simulink library "monroe_library"  (R2012b)
settings: Solver=ode45  StartTime=0.0  StopTime=10.0  RelTol=1e-3
values from neighbouring files (symbols this model uses):
  input_bit_width = ', num2str(input_bit_width))    [fft_direct_draw.m]
undefined symbols (not defined in the file or in its folder): gcbh, xlBlockLoadCallback
libraries: xbsIndex_r4 x1880, monroe_library x159, casper_library x13, xps_library x1
(part 9 of 43)

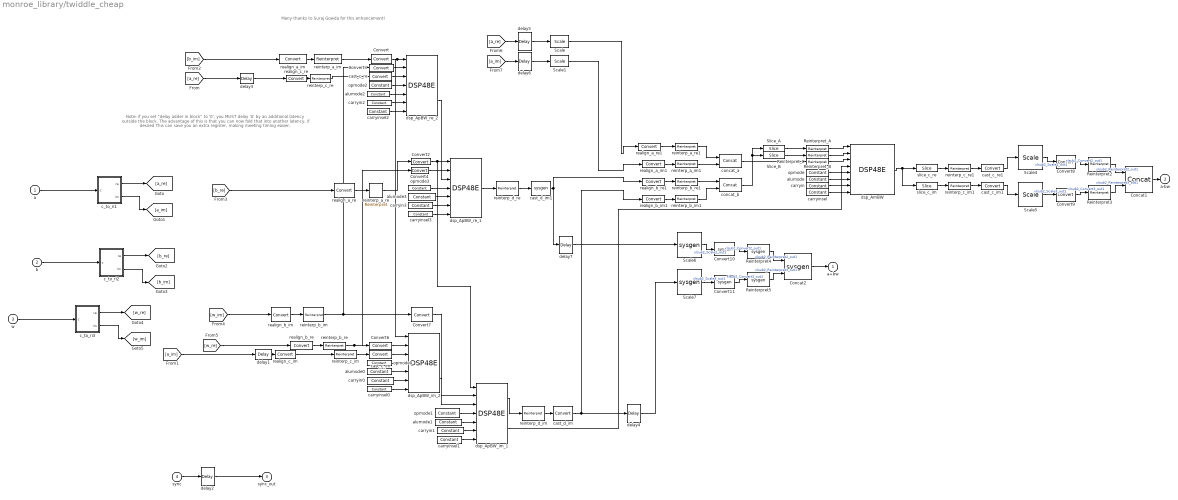
== system monroe_library/twiddle_cheap ==
  note: Note: if you set "delay adder in block" to '0', you MUST
      | delay 'A' by an additional latency outside the block.  The advantage of this
      | is that you can now fold that into another latency, if desired
      | This can save you an extra register, making meeting timing easier.
  note: Many thanks to Suraj Gowda for this enhancement!
  a : Inport
  b : Inport  Port=2
  w : Inport  Port=3
  sync : Inport  Port=4
  Concat1 : xbsIndex_r4/Concat  num_inputs=2  dbl_ovrd=off  block_type=concat
  Concat2 : S-Function  LoadFcn=xlBlockLoadCallback(gcbh);  FunctionName=sysgen  Parameters=ptable_  EnableBusSupport=off  mask(Xilinx Bus Concatenator Block){infoedit=Concatenates two or more inputs.  Output will be cast to an unsigned value with the binary point at zero., num_inputs=2, dbl_ovrd_sgadvanced=, dbl_ovrd=off, has_advanced_control=0, sggui_pos=-1,-1,-1,-1, block_type=concat, block_version=, sg_icon_stat=60,60,2,1,white,blue,0,16398980,right,,[ ],[ ], sg_mask_display=|, sg_list_contents=, sg_blockgui_xml=}
      mask sg_mask_display=|
      | fprintf('','COMMENT: begin icon graphics');
      | patch([0 60 60 0 0 ],[0 0 60 60 0 ],[0.77 0.82 0.91 ]);
      | plot([0 60 60 0 0 ],[0 0 60 60 0 ]);
      | patch([12.2 23.76 31.76 39.76 47.76 31.76 20.2 12.2 ],[38.88 38.88 46.88 38.88 46.88 46.88 46.88 38.88 ],[1 1 1 ]);
      | patch([20.2 31.76 23.76 12.2 20.2 ],[30.88 30.88 38.88 38.88 30.88 ],[0.931 0.946 0.973 ]);
      | patch([12.2 23.76 31.76 20.2 12.2 ],[22.88 22.88 30.88 30.88 22.88 ],[1 1 1 ]);
      | patch([20.2 47.76 39.76 31.76 23.76 12.2 20.2 ],[14.88 14.88 22.88 14.88 22.88 22.88 14.88 ],[0.931 0.946 0.973 ]);
      | fprintf('','COMMENT: end icon graphics');
      | fprintf('','COMMENT: begin icon text');
      | color('black');port_label('input',1,'hi');
      | color('black');port_label('input',2,'lo');
      |
      | color('black');disp('\fontsize{20}\}','texmode','on');
      | fprintf('','COMMENT: end icon text');
      mask prompts: infoedit ""; num_inputs "Number of inputs"; dbl_ovrd_sgadvanced ""; dbl_ovrd "Override with doubles"; has_advanced_control ""; sggui_pos ""; block_type ""; block_version ""; sg_icon_stat ""; sg_mask_display ""; sg_list_contents ""; sg_blockgui_xml ""
      mask help: Concatenates two or more inputs. Output will be cast to an unsigned value with the binary point at zero.
      mask init: same as monroe_library/double_delay_bram_external_counter/Concat1
      settings: CopyFcn=xlBlockMoveCallback(gcbh);  DeleteFcn=xlDestroyGui(gcbh);  ModelCloseFcn=xlDestroyGui(gcbh);  PreSaveFcn=xlBlockPreSaveCallback(gcbh);  PostSaveFcn=xlBlockPostSaveCallback(gcbh);  DestroyFcn=xlDestroyGui(gcbh);  OpenFcn=xlOpenGui(gcbh, 'concat_gui.xml', @xlmagicenablement, -1)  CloseFcn=xlDestroyGui(gcbh);  MoveFcn=xlBlockMoveCallback(gcbh);
      mask Help: eval('');xlDoc('-book','sysgen','-topic','Concat');
      mask Display:
      | fprintf('','COMMENT: begin icon graphics');
      | patch([0 60 60 0 0 ],[0 0 60 60 0 ],[0.77 0.82 0.91 ]);
      | plot([0 60 60 0 0 ],[0 0 60 60 0 ]);
      | patch([12.2 23.76 31.76 39.76 47.76 31.76 20.2 12.2 ],[38.88 38.88 46.88 38.88 46.88 46.88 46.88 38.88 ],[1 1 1 ]);
      | patch([20.2 31.76 23.76 12.2 20.2 ],[30.88 30.88 38.88 38.88 30.88 ],[0.931 0.946 0.973 ]);
      | patch([12.2 23.76 31.76 20.2 12.2 ],[22.88 22.88 30.88 30.88 22.88 ],[1 1 1 ]);
      | patch([20.2 47.76 39.76 31.76 23.76 12.2 20.2 ],[14.88 14.88 22.88 14.88 22.88 22.88 14.88 ],[0.931 0.946 0.973 ]);
      | fprintf('','COMMENT: end icon graphics');
      | fprintf('','COMMENT: begin icon text');
      | color('black');port_label('input',1,'hi');
      | color('black');port_label('input',2,'lo');
      | 
      | color('black');disp('\fontsize{20}\}','texmode','on');
      | fprintf('','COMMENT: end icon text');
  Convert : xbsIndex_r4/Convert  arith_type="Signed  (2's comp)"  n_bits=30  bin_pt=0  quantization=Truncate  overflow=Wrap  en=off  latency=0  dbl_ovrd=off  pipeline=on  block_type=convert
      settings: block_version=11.4
  Convert10 : S-Function  LoadFcn=xlBlockLoadCallback(gcbh);  FunctionName=sysgen  Parameters=ptable_  EnableBusSupport=off  mask(Xilinx Type Converter Block){infoedit=Hardware notes: rounding and saturating require hardware resources; truncating and wrapping do not., arith_type_sgadvanced=, arith_type=Signed  (2's comp), n_bits=out_n_bits, bin_pt=out_n_bits-1, quantization_sgadvanced=, quantization=Truncate, overflow_sgadvanced=, overflow=Wrap, en_sgadvanced=, en=off, latency=0, dbl_ovrd_sgadvanced=, dbl_ovrd=off, pipeline_sgadvanced=, pipeline=off, xl_use_area_sgadvanced=, xl_use_area=off, xl_area=[0,0,0,0,0,0,0], has_advanced_control=0, sggui_pos=-1,-1,-1,-1, block_type=convert, block_version=, sg_icon_stat=45,30,1,1,white,blue,0,edca21da,right,,[ ],[ ], sg_mask_display=|, sg_list_contents=, sg_blockgui_xml=}
      mask sg_mask_display=|
      | fprintf('','COMMENT: begin icon graphics');
      | patch([0 45 45 0 0 ],[0 0 30 30 0 ],[0.77 0.82 0.91 ]);
      | plot([0 45 45 0 0 ],[0 0 30 30 0 ]);
      | patch([13.1 18.88 22.88 26.88 30.88 22.88 17.1 13.1 ],[19.44 19.44 23.44 19.44 23.44 23.44 23.44 19.44 ],[1 1 1 ]);
      | patch([17.1 22.88 18.88 13.1 17.1 ],[15.44 15.44 19.44 19.44 15.44 ],[0.931 0.946 0.973 ]);
      | patch([13.1 18.88 22.88 17.1 13.1 ],[11.44 11.44 15.44 15.44 11.44 ],[1 1 1 ]);
      | patch([17.1 30.88 26.88 22.88 18.88 13.1 17.1 ],[7.44 7.44 11.44 7.44 11.44 11.44 7.44 ],[0.931 0.946 0.973 ]);
      | fprintf('','COMMENT: end icon graphics');
      | fprintf('','COMMENT: begin icon text');
      |
      | color('black');port_label('output',1,'cast');
      | fprintf('','COMMENT: end icon text');
      mask prompts: infoedit ""; arith_type_sgadvanced ""; arith_type "Type"; n_bits "Number of bits"; bin_pt "Binary point"; quantization_sgadvanced ""; overflow_sgadvanced ""; en_sgadvanced ""; en "Provide enable port"; dbl_ovrd_sgadvanced ""; dbl_ovrd "Override with doubles"; pipeline_sgadvanced ""; pipeline "Pipeline for maximum performance"; xl_use_area_sgadvanced ""; xl_use_area "Define FPGA area for resource estimation"; xl_area "FPGA area [slices, FFs, BRAMs, LUTs, IOBs, emb. mults, TBUFs]"; has_advanced_control ""; sggui_pos ""; block_type ""; block_version ""; sg_icon_stat ""; sg_mask_display ""; sg_list_contents ""; sg_blockgui_xml ""
      mask help: Hardware notes: rounding and saturating require hardware resources; truncating and wrapping do not.
      mask init: same as monroe_library/dsp48e_mult_add_pcin/Convert
      settings: CopyFcn=xlBlockMoveCallback(gcbh);  DeleteFcn=xlDestroyGui(gcbh);  ModelCloseFcn=xlDestroyGui(gcbh);  PreSaveFcn=xlBlockPreSaveCallback(gcbh);  PostSaveFcn=xlBlockPostSaveCallback(gcbh);  DestroyFcn=xlDestroyGui(gcbh);  OpenFcn=xlOpenGui(gcbh, 'convert_gui.xml', @convertenablement, -1)  CloseFcn=xlDestroyGui(gcbh);  MoveFcn=xlBlockMoveCallback(gcbh);
      mask Help: eval('');xlDoc('-book','sysgen','-topic','Convert');
      mask TypeOptions arith_type: Boolean | Signed  (2's comp) | Unsigned
      mask TypeOptions quantization: Truncate | Round  (unbiased: +/- Inf) | Round  (unbiased: Even Values)
      mask TypeOptions overflow: Wrap | Saturate | Flag as error
      mask Display:
      | fprintf('','COMMENT: begin icon graphics');
      | patch([0 45 45 0 0 ],[0 0 30 30 0 ],[0.77 0.82 0.91 ]);
      | plot([0 45 45 0 0 ],[0 0 30 30 0 ]);
      | patch([13.1 18.88 22.88 26.88 30.88 22.88 17.1 13.1 ],[19.44 19.44 23.44 19.44 23.44 23.44 23.44 19.44 ],[1 1 1 ]);
      | patch([17.1 22.88 18.88 13.1 17.1 ],[15.44 15.44 19.44 19.44 15.44 ],[0.931 0.946 0.973 ]);
      | patch([13.1 18.88 22.88 17.1 13.1 ],[11.44 11.44 15.44 15.44 11.44 ],[1 1 1 ]);
      | patch([17.1 30.88 26.88 22.88 18.88 13.1 17.1 ],[7.44 7.44 11.44 7.44 11.44 11.44 7.44 ],[0.931 0.946 0.973 ]);
      | fprintf('','COMMENT: end icon graphics');
      | fprintf('','COMMENT: begin icon text');
      | 
      | color('black');port_label('output',1,'cast');
      | fprintf('','COMMENT: end icon text');
  Convert11 : S-Function  LoadFcn=xlBlockLoadCallback(gcbh);  FunctionName=sysgen  Parameters=ptable_  EnableBusSupport=off  mask(Xilinx Type Converter Block){infoedit=Hardware notes: rounding and saturating require hardware resources; truncating and wrapping do not., arith_type_sgadvanced=, arith_type=Signed  (2's comp), n_bits=out_n_bits, bin_pt=out_n_bits-1, quantization_sgadvanced=, quantization=Truncate, overflow_sgadvanced=, overflow=Wrap, en_sgadvanced=, en=off, latency=0, dbl_ovrd_sgadvanced=, dbl_ovrd=off, pipeline_sgadvanced=, pipeline=off, xl_use_area_sgadvanced=, xl_use_area=off, xl_area=[0,0,0,0,0,0,0], has_advanced_control=0, sggui_pos=-1,-1,-1,-1, block_type=convert, block_version=, sg_icon_stat=45,30,1,1,white,blue,0,edca21da,right,,[ ],[ ], sg_mask_display=|, sg_list_contents=, sg_blockgui_xml=}
      mask sg_mask_display=|
      | fprintf('','COMMENT: begin icon graphics');
      | patch([0 45 45 0 0 ],[0 0 30 30 0 ],[0.77 0.82 0.91 ]);
      | plot([0 45 45 0 0 ],[0 0 30 30 0 ]);
      | patch([13.1 18.88 22.88 26.88 30.88 22.88 17.1 13.1 ],[19.44 19.44 23.44 19.44 23.44 23.44 23.44 19.44 ],[1 1 1 ]);
      | patch([17.1 22.88 18.88 13.1 17.1 ],[15.44 15.44 19.44 19.44 15.44 ],[0.931 0.946 0.973 ]);
      | patch([13.1 18.88 22.88 17.1 13.1 ],[11.44 11.44 15.44 15.44 11.44 ],[1 1 1 ]);
      | patch([17.1 30.88 26.88 22.88 18.88 13.1 17.1 ],[7.44 7.44 11.44 7.44 11.44 11.44 7.44 ],[0.931 0.946 0.973 ]);
      | fprintf('','COMMENT: end icon graphics');
      | fprintf('','COMMENT: begin icon text');
      |
      | color('black');port_label('output',1,'cast');
      | fprintf('','COMMENT: end icon text');
      mask prompts: infoedit ""; arith_type_sgadvanced ""; arith_type "Type"; n_bits "Number of bits"; bin_pt "Binary point"; quantization_sgadvanced ""; overflow_sgadvanced ""; en_sgadvanced ""; en "Provide enable port"; dbl_ovrd_sgadvanced ""; dbl_ovrd "Override with doubles"; pipeline_sgadvanced ""; pipeline "Pipeline for maximum performance"; xl_use_area_sgadvanced ""; xl_use_area "Define FPGA area for resource estimation"; xl_area "FPGA area [slices, FFs, BRAMs, LUTs, IOBs, emb. mults, TBUFs]"; has_advanced_control ""; sggui_pos ""; block_type ""; block_version ""; sg_icon_stat ""; sg_mask_display ""; sg_list_contents ""; sg_blockgui_xml ""
      mask help: Hardware notes: rounding and saturating require hardware resources; truncating and wrapping do not.
      mask init: same as monroe_library/dsp48e_mult_add_pcin/Convert
      settings: CopyFcn=xlBlockMoveCallback(gcbh);  DeleteFcn=xlDestroyGui(gcbh);  ModelCloseFcn=xlDestroyGui(gcbh);  PreSaveFcn=xlBlockPreSaveCallback(gcbh);  PostSaveFcn=xlBlockPostSaveCallback(gcbh);  DestroyFcn=xlDestroyGui(gcbh);  OpenFcn=xlOpenGui(gcbh, 'convert_gui.xml', @convertenablement, -1)  CloseFcn=xlDestroyGui(gcbh);  MoveFcn=xlBlockMoveCallback(gcbh);
      mask Help: eval('');xlDoc('-book','sysgen','-topic','Convert');
      mask TypeOptions arith_type: Boolean | Signed  (2's comp) | Unsigned
      mask TypeOptions quantization: Truncate | Round  (unbiased: +/- Inf) | Round  (unbiased: Even Values)
      mask TypeOptions overflow: Wrap | Saturate | Flag as error
      mask Display:
      | fprintf('','COMMENT: begin icon graphics');
      | patch([0 45 45 0 0 ],[0 0 30 30 0 ],[0.77 0.82 0.91 ]);
      | plot([0 45 45 0 0 ],[0 0 30 30 0 ]);
      | patch([13.1 18.88 22.88 26.88 30.88 22.88 17.1 13.1 ],[19.44 19.44 23.44 19.44 23.44 23.44 23.44 19.44 ],[1 1 1 ]);
      | patch([17.1 22.88 18.88 13.1 17.1 ],[15.44 15.44 19.44 19.44 15.44 ],[0.931 0.946 0.973 ]);
      | patch([13.1 18.88 22.88 17.1 13.1 ],[11.44 11.44 15.44 15.44 11.44 ],[1 1 1 ]);
      | patch([17.1 30.88 26.88 22.88 18.88 13.1 17.1 ],[7.44 7.44 11.44 7.44 11.44 11.44 7.44 ],[0.931 0.946 0.973 ]);
      | fprintf('','COMMENT: end icon graphics');
      | fprintf('','COMMENT: begin icon text');
      | 
      | color('black');port_label('output',1,'cast');
      | fprintf('','COMMENT: end icon text');
  Convert2 : xbsIndex_r4/Convert  arith_type="Signed  (2's comp)"  n_bits=30  bin_pt=0  quantization=Truncate  overflow=Wrap  en=off  latency=0  dbl_ovrd=off  pipeline=on  block_type=convert
      settings: block_version=11.4
  Convert{3..4,6..7} (4 alike) : xbsIndex_r4/Convert  arith_type="Signed  (2's comp)"  n_bits=18  bin_pt=0  quantization=Truncate  overflow=Wrap  en=off  latency=0  dbl_ovrd=off  pipeline=on  block_type=convert
      settings: block_version=11.4
  Convert8 : xbsIndex_r4/Convert  arith_type="Signed  (2's comp)"  n_bits=out_n_bits  bin_pt=out_n_bits-1  quantization=Truncate  overflow=Wrap  en=off  latency=0  dbl_ovrd=off  pipeline=off  block_type=convert
  Convert9 : xbsIndex_r4/Convert  arith_type="Signed  (2's comp)"  n_bits=out_n_bits  bin_pt=out_n_bits-1  quantization=Truncate  overflow=Wrap  en=off  latency=0  dbl_ovrd=off  pipeline=off  block_type=convert
  Reinterpret2 : xbsIndex_r4/Reinterpret  force_arith_type=on  arith_type=Unsigned  force_bin_pt=on  bin_pt=0  block_type=reinterpret
      settings: infoedit="Changes signal type without altering the binary representation.   You can changed the signal between signed and unsigned, and relocate the binary point.<br><br>Hardware notes: In hardware this block costs nothing.<br><br>Example:  Suppose the input is 6 bits wide, signed, with 2 fractional bits, and the output is forced to unsigned with 0 fractional bits.  Then an input of -2.0 (1110.00 in binary 2's complement) becomes an output of 56 (111000 in binary)."
  Reinterpret3 : xbsIndex_r4/Reinterpret  force_arith_type=on  arith_type=Unsigned  force_bin_pt=on  bin_pt=0  block_type=reinterpret
      settings: infoedit="Changes signal type without altering the binary representation.   You can changed the signal between signed and unsigned, and relocate the binary point.<br><br>Hardware notes: In hardware this block costs nothing.<br><br>Example:  Suppose the input is 6 bits wide, signed, with 2 fractional bits, and the output is forced to unsigned with 0 fractional bits.  Then an input of -2.0 (1110.00 in binary 2's complement) becomes an output of 56 (111000 in binary)."
  Reinterpret4 : S-Function  LoadFcn=xlBlockLoadCallback(gcbh);  FunctionName=sysgen  Parameters=ptable_  EnableBusSupport=off  mask(Xilinx Type Reinterpreter Block){infoedit=Changes signal type without altering the binary representation.   You can changed the signal between signed and unsigned, and relocate the binary point.<br><br>Hardware notes: In hardware this block costs nothing.<br><br>Example:  Suppose the input is 6 bits wide, signed, with 2 fractional bits, and the output is forced to unsigned with 0 fractional bits.  Then an input of -2.0 (1110.00 in binary 2's complement) becomes an output of 56 (111000 in binary)., force_arith_type_sgadvanced=, force_arith_type=on, arith_type_sgadvanced=, arith_type=Unsigned, force_bin_pt_sgadvanced=, force_bin_pt=on, bin_pt=0, has_advanced_control=0, sggui_pos=-1,-1,-1,-1, block_type=reinterpret, block_version=, sg_icon_stat=50,32,1,1,white,blue,0,6b04d0b0,right,,[ ],[ ], sg_mask_display=|, sg_list_contents=, sg_blockgui_xml=}
      mask sg_mask_display=|
      | fprintf('','COMMENT: begin icon graphics');
      | patch([0 50 50 0 0 ],[0 0 32 32 0 ],[0.77 0.82 0.91 ]);
      | plot([0 50 50 0 0 ],[0 0 32 32 0 ]);
      | patch([16.1 21.88 25.88 29.88 33.88 25.88 20.1 16.1 ],[20.44 20.44 24.44 20.44 24.44 24.44 24.44 20.44 ],[1 1 1 ]);
      | patch([20.1 25.88 21.88 16.1 20.1 ],[16.44 16.44 20.44 20.44 16.44 ],[0.931 0.946 0.973 ]);
      | patch([16.1 21.88 25.88 20.1 16.1 ],[12.44 12.44 16.44 16.44 12.44 ],[1 1 1 ]);
      | patch([20.1 33.88 29.88 25.88 21.88 16.1 20.1 ],[8.44 8.44 12.44 8.44 12.44 12.44 8.44 ],[0.931 0.946 0.973 ]);
      | fprintf('','COMMENT: end icon graphics');
      | fprintf('','COMMENT: begin icon text');
      |
      |
      | color('black');disp('reinterpret');
      | fprintf('','COMMENT: end icon text');
      mask prompts: infoedit ""; force_arith_type_sgadvanced ""; force_arith_type "Force Arithmetic Type"; arith_type_sgadvanced ""; arith_type "Output Arithmetic Type"; force_bin_pt_sgadvanced ""; force_bin_pt "Force Binary Point"; bin_pt "Output Binary Point"; has_advanced_control ""; sggui_pos ""; block_type ""; block_version ""; sg_icon_stat ""; sg_mask_display ""; sg_list_contents ""; sg_blockgui_xml ""
      mask help:
      | Changes signal type without altering the binary representation.   You can changed the signal between signed and unsigned, and relocate the binary point.
      |
      | Hardware notes: In hardware this block costs nothing.
      |
      | Example:  Suppose the input is 6 bits wide, signed, with 2 fractional bits, and the output is forced to unsigned with 0 fractional bits.  Then an input of -2.0 (1110.00 in binary 2's complement) becomes an output of 56 (111000 in binary).
      mask init:
      | try
      |   tmp_gcb = gcb;
      |   tmp_gcbh = gcbh;
      |   if (strcmp('SysGenIndex',get_param(bdroot(tmp_gcbh),'tag')) && ~isempty(regexp(bdroot(tmp_gcb), '^xbs', 'once')))
      |     return;
      |   end;
      |   xlMungeMaskParams;
      |   block_config = 'sysgen_blockset:Reinterpret_config';
      | 
      |   block_type='reinterpret';
      | 
      |   serialized_declarations = '{''arith_type''=>''Int'',''bin_pt''=>''Int'',''force_arith_type''=>''Bool'',''force_bin_pt''=>''Bool'',''block_type''=>''String''}';
      |   ptable_ = xlblockprep(get_param(tmp_gcb, 'MaskWSVariables'));
      |   try
      |     xlBlockMoveCallback(tmp_gcbh);
      |   catch 
      |      clear global xl_updateicon_recursion_guard;
      |   end;
      | catch
      |   global dbgsysgen;
      |   if(~isempty(dbgsysgen) && dbgsysgen)
      |     e = regexprep(lasterr, '\n', '\nError: ');
      |     disp(['Error: While running MaskInit code on block ' tmp_gcb ': ' e]);
      |     error(e);
      |   end
      | end
      settings: CopyFcn=xlBlockMoveCallback(gcbh);  DeleteFcn=xlDestroyGui(gcbh);  ModelCloseFcn=xlDestroyGui(gcbh);  PreSaveFcn=xlBlockPreSaveCallback(gcbh);  PostSaveFcn=xlBlockPostSaveCallback(gcbh);  DestroyFcn=xlDestroyGui(gcbh);  OpenFcn=xlOpenGui(gcbh, 'reinterpret_gui.xml', @reinterpretenablement, -1)  CloseFcn=xlDestroyGui(gcbh);  MoveFcn=xlBlockMoveCallback(gcbh);
      mask Help: eval('');xlDoc('-book','sysgen','-topic','Reinterpret');
      mask TypeOptions arith_type: Unsigned | Signed  (2's comp)
      mask Display:
      | fprintf('','COMMENT: begin icon graphics');
      | patch([0 50 50 0 0 ],[0 0 32 32 0 ],[0.77 0.82 0.91 ]);
      | plot([0 50 50 0 0 ],[0 0 32 32 0 ]);
      | patch([16.1 21.88 25.88 29.88 33.88 25.88 20.1 16.1 ],[20.44 20.44 24.44 20.44 24.44 24.44 24.44 20.44 ],[1 1 1 ]);
      | patch([20.1 25.88 21.88 16.1 20.1 ],[16.44 16.44 20.44 20.44 16.44 ],[0.931 0.946 0.973 ]);
      | patch([16.1 21.88 25.88 20.1 16.1 ],[12.44 12.44 16.44 16.44 12.44 ],[1 1 1 ]);
      | patch([20.1 33.88 29.88 25.88 21.88 16.1 20.1 ],[8.44 8.44 12.44 8.44 12.44 12.44 8.44 ],[0.931 0.946 0.973 ]);
      | fprintf('','COMMENT: end icon graphics');
      | fprintf('','COMMENT: begin icon text');
      | 
      | 
      | color('black');disp('reinterpret');
      | fprintf('','COMMENT: end icon text');
  Reinterpret5 : S-Function  LoadFcn=xlBlockLoadCallback(gcbh);  FunctionName=sysgen  Parameters=ptable_  EnableBusSupport=off  mask(Xilinx Type Reinterpreter Block){infoedit=Changes signal type without altering the binary representation.   You can changed the signal between signed and unsigned, and relocate the binary point.<br><br>Hardware notes: In hardware this block costs nothing.<br><br>Example:  Suppose the input is 6 bits wide, signed, with 2 fractional bits, and the output is forced to unsigned with 0 fractional bits.  Then an input of -2.0 (1110.00 in binary 2's complement) becomes an output of 56 (111000 in binary)., force_arith_type_sgadvanced=, force_arith_type=on, arith_type_sgadvanced=, arith_type=Unsigned, force_bin_pt_sgadvanced=, force_bin_pt=on, bin_pt=0, has_advanced_control=0, sggui_pos=-1,-1,-1,-1, block_type=reinterpret, block_version=, sg_icon_stat=50,32,1,1,white,blue,0,6b04d0b0,right,,[ ],[ ], sg_mask_display=|, sg_list_contents=, sg_blockgui_xml=}
      mask sg_mask_display=|
      | fprintf('','COMMENT: begin icon graphics');
      | patch([0 50 50 0 0 ],[0 0 32 32 0 ],[0.77 0.82 0.91 ]);
      | plot([0 50 50 0 0 ],[0 0 32 32 0 ]);
      | patch([16.1 21.88 25.88 29.88 33.88 25.88 20.1 16.1 ],[20.44 20.44 24.44 20.44 24.44 24.44 24.44 20.44 ],[1 1 1 ]);
      | patch([20.1 25.88 21.88 16.1 20.1 ],[16.44 16.44 20.44 20.44 16.44 ],[0.931 0.946 0.973 ]);
      | patch([16.1 21.88 25.88 20.1 16.1 ],[12.44 12.44 16.44 16.44 12.44 ],[1 1 1 ]);
      | patch([20.1 33.88 29.88 25.88 21.88 16.1 20.1 ],[8.44 8.44 12.44 8.44 12.44 12.44 8.44 ],[0.931 0.946 0.973 ]);
      | fprintf('','COMMENT: end icon graphics');
      | fprintf('','COMMENT: begin icon text');
      |
      |
      | color('black');disp('reinterpret');
      | fprintf('','COMMENT: end icon text');
      mask prompts: infoedit ""; force_arith_type_sgadvanced ""; force_arith_type "Force Arithmetic Type"; arith_type_sgadvanced ""; arith_type "Output Arithmetic Type"; force_bin_pt_sgadvanced ""; force_bin_pt "Force Binary Point"; bin_pt "Output Binary Point"; has_advanced_control ""; sggui_pos ""; block_type ""; block_version ""; sg_icon_stat ""; sg_mask_display ""; sg_list_contents ""; sg_blockgui_xml ""
      mask help:
      | Changes signal type without altering the binary representation.   You can changed the signal between signed and unsigned, and relocate the binary point.
      |
      | Hardware notes: In hardware this block costs nothing.
      |
      | Example:  Suppose the input is 6 bits wide, signed, with 2 fractional bits, and the output is forced to unsigned with 0 fractional bits.  Then an input of -2.0 (1110.00 in binary 2's complement) becomes an output of 56 (111000 in binary).
      mask init: same as monroe_library/twiddle_cheap/Reinterpret4
      settings: CopyFcn=xlBlockMoveCallback(gcbh);  DeleteFcn=xlDestroyGui(gcbh);  ModelCloseFcn=xlDestroyGui(gcbh);  PreSaveFcn=xlBlockPreSaveCallback(gcbh);  PostSaveFcn=xlBlockPostSaveCallback(gcbh);  DestroyFcn=xlDestroyGui(gcbh);  OpenFcn=xlOpenGui(gcbh, 'reinterpret_gui.xml', @reinterpretenablement, -1)  CloseFcn=xlDestroyGui(gcbh);  MoveFcn=xlBlockMoveCallback(gcbh);
      mask Help: eval('');xlDoc('-book','sysgen','-topic','Reinterpret');
      mask TypeOptions arith_type: Unsigned | Signed  (2's comp)
      mask Display:
      | fprintf('','COMMENT: begin icon graphics');
      | patch([0 50 50 0 0 ],[0 0 32 32 0 ],[0.77 0.82 0.91 ]);
      | plot([0 50 50 0 0 ],[0 0 32 32 0 ]);
      | patch([16.1 21.88 25.88 29.88 33.88 25.88 20.1 16.1 ],[20.44 20.44 24.44 20.44 24.44 24.44 24.44 20.44 ],[1 1 1 ]);
      | patch([20.1 25.88 21.88 16.1 20.1 ],[16.44 16.44 20.44 20.44 16.44 ],[0.931 0.946 0.973 ]);
      | patch([16.1 21.88 25.88 20.1 16.1 ],[12.44 12.44 16.44 16.44 12.44 ],[1 1 1 ]);
      | patch([20.1 33.88 29.88 25.88 21.88 16.1 20.1 ],[8.44 8.44 12.44 8.44 12.44 12.44 8.44 ],[0.931 0.946 0.973 ]);
      | fprintf('','COMMENT: end icon graphics');
      | fprintf('','COMMENT: begin icon text');
      | 
      | 
      | color('black');disp('reinterpret');
      | fprintf('','COMMENT: end icon text');
  Reinterpret_A : xbsIndex_r4/Reinterpret  force_arith_type=on  arith_type="Signed  (2's comp)"  force_bin_pt=on  bin_pt=0  block_type=reinterpret
      settings: infoedit="Changes signal type without altering the binary representation.   You can changed the signal between signed and unsigned, and relocate the binary point.<br><br>Hardware notes: In hardware this block costs nothing.<br><br>Example:  Suppose the input is 6 bits wide, signed, with 2 fractional bits, and the output is forced to unsigned with 0 fractional bits.  Then an input of -2.0 (1110.00 in binary 2's complement) becomes an output of 56 (111000 in binary)."  block_version=10.1.3
  Reinterpret_B : xbsIndex_r4/Reinterpret  force_arith_type=on  arith_type="Signed  (2's comp)"  force_bin_pt=on  bin_pt=0  block_type=reinterpret
      settings: infoedit="Changes signal type without altering the binary representation.   You can changed the signal between signed and unsigned, and relocate the binary point.<br><br>Hardware notes: In hardware this block costs nothing.<br><br>Example:  Suppose the input is 6 bits wide, signed, with 2 fractional bits, and the output is forced to unsigned with 0 fractional bits.  Then an input of -2.0 (1110.00 in binary 2's complement) becomes an output of 56 (111000 in binary)."  block_version=10.1.3
  Reinterpret_C : xbsIndex_r4/Reinterpret  force_arith_type=on  arith_type="Signed  (2's comp)"  force_bin_pt=on  bin_pt=0  block_type=reinterpret
      settings: infoedit="Changes signal type without altering the binary representation.   You can changed the signal between signed and unsigned, and relocate the binary point.<br><br>Hardware notes: In hardware this block costs nothing.<br><br>Example:  Suppose the input is 6 bits wide, signed, with 2 fractional bits, and the output is forced to unsigned with 0 fractional bits.  Then an input of -2.0 (1110.00 in binary 2's complement) becomes an output of 56 (111000 in binary)."  block_version=10.1.3
  Scale : xbsIndex_r4/Scale  scale_factor=1  dbl_ovrd=off  block_type=scale
  Scale1 : xbsIndex_r4/Scale  scale_factor=1  dbl_ovrd=off  block_type=scale
  Scale4 : xbsIndex_r4/Scale  scale_factor=downshift_at_end*-1  dbl_ovrd=off  block_type=scale
  Scale5 : xbsIndex_r4/Scale  scale_factor=downshift_at_end*-1  dbl_ovrd=off  block_type=scale
  Scale6 : S-Function  LoadFcn=xlBlockLoadCallback(gcbh);  FunctionName=sysgen  Parameters=ptable_  EnableBusSupport=off  mask(Xilinx Input Scaler Block){infoedit=Scales input by a power of two by adjusting the binary point position.<br><br>Hardware notes: In hardware this block costs nothing., scale_factor=downshift_at_end*-1, dbl_ovrd_sgadvanced=, dbl_ovrd=off, has_advanced_control=0, sggui_pos=-1,-1,-1,-1, block_type=scale, block_version=, sg_icon_stat=55,56,1,1,white,blue,0,e7f93c29,right,,[ ],[ ], sg_mask_display=|, sg_list_contents=, sg_blockgui_xml=}
      mask sg_mask_display=|
      | fprintf('','COMMENT: begin icon graphics');
      | patch([0 55 55 0 0 ],[0 0 56 56 0 ],[0.77 0.82 0.91 ]);
      | plot([0 55 55 0 0 ],[0 0 56 56 0 ]);
      | patch([11.425 21.54 28.54 35.54 42.54 28.54 18.425 11.425 ],[35.77 35.77 42.77 35.77 42.77 42.77 42.77 35.77 ],[1 1 1 ]);
      | patch([18.425 28.54 21.54 11.425 18.425 ],[28.77 28.77 35.77 35.77 28.77 ],[0.931 0.946 0.973 ]);
      | patch([11.425 21.54 28.54 18.425 11.425 ],[21.77 21.77 28.77 28.77 21.77 ],[1 1 1 ]);
      | patch([18.425 42.54 35.54 28.54 21.54 11.425 18.425 ],[14.77 14.77 21.77 14.77 21.77 21.77 14.77 ],[0.931 0.946 0.973 ]);
      | fprintf('','COMMENT: end icon graphics');
      | fprintf('','COMMENT: begin icon text');
      |
      |
      | color('black');disp('\bf{2^{0}}','texmode','on');
      | fprintf('','COMMENT: end icon text');
      mask prompts: infoedit ""; scale_factor "Scale factor s (scale output by 2^s)"; dbl_ovrd_sgadvanced ""; dbl_ovrd "Override with doubles"; has_advanced_control ""; sggui_pos ""; block_type ""; block_version ""; sg_icon_stat ""; sg_mask_display ""; sg_list_contents ""; sg_blockgui_xml ""
      mask help:
      | Scales input by a power of two by adjusting the binary point position.
      |
      | Hardware notes: In hardware this block costs nothing.
      mask init:
      | try
      |   tmp_gcb = gcb;
      |   tmp_gcbh = gcbh;
      |   if (strcmp('SysGenIndex',get_param(bdroot(tmp_gcbh),'tag')) && ~isempty(regexp(bdroot(tmp_gcb), '^xbs', 'once')))
      |     return;
      |   end;
      |   xlMungeMaskParams;
      |   block_config = 'sysgen_blockset:Scale_config';
      | 
      |   block_type='scale';
      | 
      |   serialized_declarations = '{''dbl_ovrd''=>''Int'',''scale_factor''=>''Int'',''block_type''=>''String''}';
      |   xlscale_init();
      |   ptable_ = xlblockprep(get_param(tmp_gcb, 'MaskWSVariables'));
      |   try
      |     xlBlockMoveCallback(tmp_gcbh);
      |   catch 
      |      clear global xl_updateicon_recursion_guard;
      |   end;
      | catch
      |   global dbgsysgen;
      |   if(~isempty(dbgsysgen) && dbgsysgen)
      |     e = regexprep(lasterr, '\n', '\nError: ');
      |     disp(['Error: While running MaskInit code on block ' tmp_gcb ': ' e]);
      |     error(e);
      |   end
      | end
      settings: CopyFcn=xlBlockMoveCallback(gcbh);  DeleteFcn=xlDestroyGui(gcbh);  ModelCloseFcn=xlDestroyGui(gcbh);  PreSaveFcn=xlBlockPreSaveCallback(gcbh);  PostSaveFcn=xlBlockPostSaveCallback(gcbh);  DestroyFcn=xlDestroyGui(gcbh);  OpenFcn=xlOpenGui(gcbh, 'scale_gui.xml', @xlmagicenablement, -1)  CloseFcn=xlDestroyGui(gcbh);  MoveFcn=xlBlockMoveCallback(gcbh);
      mask Help: eval('');xlDoc('-book','sysgen','-topic','Scale');
      mask Display:
      | fprintf('','COMMENT: begin icon graphics');
      | patch([0 55 55 0 0 ],[0 0 56 56 0 ],[0.77 0.82 0.91 ]);
      | plot([0 55 55 0 0 ],[0 0 56 56 0 ]);
      | patch([11.425 21.54 28.54 35.54 42.54 28.54 18.425 11.425 ],[35.77 35.77 42.77 35.77 42.77 42.77 42.77 35.77 ],[1 1 1 ]);
      | patch([18.425 28.54 21.54 11.425 18.425 ],[28.77 28.77 35.77 35.77 28.77 ],[0.931 0.946 0.973 ]);
      | patch([11.425 21.54 28.54 18.425 11.425 ],[21.77 21.77 28.77 28.77 21.77 ],[1 1 1 ]);
      | patch([18.425 42.54 35.54 28.54 21.54 11.425 18.425 ],[14.77 14.77 21.77 14.77 21.77 21.77 14.77 ],[0.931 0.946 0.973 ]);
      | fprintf('','COMMENT: end icon graphics');
      | fprintf('','COMMENT: begin icon text');
      | 
      | 
      | color('black');disp('\bf{2^{0}}','texmode','on');
      | fprintf('','COMMENT: end icon text');
  Scale7 : S-Function  LoadFcn=xlBlockLoadCallback(gcbh);  FunctionName=sysgen  Parameters=ptable_  EnableBusSupport=off  mask(Xilinx Input Scaler Block){infoedit=Scales input by a power of two by adjusting the binary point position.<br><br>Hardware notes: In hardware this block costs nothing., scale_factor=downshift_at_end*-1, dbl_ovrd_sgadvanced=, dbl_ovrd=off, has_advanced_control=0, sggui_pos=-1,-1,-1,-1, block_type=scale, block_version=, sg_icon_stat=55,56,1,1,white,blue,0,e7f93c29,right,,[ ],[ ], sg_mask_display=|, sg_list_contents=, sg_blockgui_xml=}
      mask sg_mask_display=|
      | fprintf('','COMMENT: begin icon graphics');
      | patch([0 55 55 0 0 ],[0 0 56 56 0 ],[0.77 0.82 0.91 ]);
      | plot([0 55 55 0 0 ],[0 0 56 56 0 ]);
      | patch([11.425 21.54 28.54 35.54 42.54 28.54 18.425 11.425 ],[35.77 35.77 42.77 35.77 42.77 42.77 42.77 35.77 ],[1 1 1 ]);
      | patch([18.425 28.54 21.54 11.425 18.425 ],[28.77 28.77 35.77 35.77 28.77 ],[0.931 0.946 0.973 ]);
      | patch([11.425 21.54 28.54 18.425 11.425 ],[21.77 21.77 28.77 28.77 21.77 ],[1 1 1 ]);
      | patch([18.425 42.54 35.54 28.54 21.54 11.425 18.425 ],[14.77 14.77 21.77 14.77 21.77 21.77 14.77 ],[0.931 0.946 0.973 ]);
      | fprintf('','COMMENT: end icon graphics');
      | fprintf('','COMMENT: begin icon text');
      |
      |
      | color('black');disp('\bf{2^{0}}','texmode','on');
      | fprintf('','COMMENT: end icon text');
      mask prompts: infoedit ""; scale_factor "Scale factor s (scale output by 2^s)"; dbl_ovrd_sgadvanced ""; dbl_ovrd "Override with doubles"; has_advanced_control ""; sggui_pos ""; block_type ""; block_version ""; sg_icon_stat ""; sg_mask_display ""; sg_list_contents ""; sg_blockgui_xml ""
      mask help:
      | Scales input by a power of two by adjusting the binary point position.
      |
      | Hardware notes: In hardware this block costs nothing.
      mask init: same as monroe_library/twiddle_cheap/Scale6
      settings: CopyFcn=xlBlockMoveCallback(gcbh);  DeleteFcn=xlDestroyGui(gcbh);  ModelCloseFcn=xlDestroyGui(gcbh);  PreSaveFcn=xlBlockPreSaveCallback(gcbh);  PostSaveFcn=xlBlockPostSaveCallback(gcbh);  DestroyFcn=xlDestroyGui(gcbh);  OpenFcn=xlOpenGui(gcbh, 'scale_gui.xml', @xlmagicenablement, -1)  CloseFcn=xlDestroyGui(gcbh);  MoveFcn=xlBlockMoveCallback(gcbh);
      mask Help: eval('');xlDoc('-book','sysgen','-topic','Scale');
      mask Display:
      | fprintf('','COMMENT: begin icon graphics');
      | patch([0 55 55 0 0 ],[0 0 56 56 0 ],[0.77 0.82 0.91 ]);
      | plot([0 55 55 0 0 ],[0 0 56 56 0 ]);
      | patch([11.425 21.54 28.54 35.54 42.54 28.54 18.425 11.425 ],[35.77 35.77 42.77 35.77 42.77 42.77 42.77 35.77 ],[1 1 1 ]);
      | patch([18.425 28.54 21.54 11.425 18.425 ],[28.77 28.77 35.77 35.77 28.77 ],[0.931 0.946 0.973 ]);
      | patch([11.425 21.54 28.54 18.425 11.425 ],[21.77 21.77 28.77 28.77 21.77 ],[1 1 1 ]);
      | patch([18.425 42.54 35.54 28.54 21.54 11.425 18.425 ],[14.77 14.77 21.77 14.77 21.77 21.77 14.77 ],[0.931 0.946 0.973 ]);
      | fprintf('','COMMENT: end icon graphics');
      | fprintf('','COMMENT: begin icon text');
      | 
      | 
      | color('black');disp('\bf{2^{0}}','texmode','on');
      | fprintf('','COMMENT: end icon text');
  Slice_A : xbsIndex_r4/Slice  nbits=30  boolean_output=off  mode=Upper Bit Location + Width  bit1=0  base1=MSB of Input  bit0=0  base0=LSB of Input  dbl_ovrd=off  block_type=slice
  Slice_B : xbsIndex_r4/Slice  nbits=18  boolean_output=off  mode=Lower Bit Location + Width  bit1=0  base1=MSB of Input  bit0=0  base0=LSB of Input  dbl_ovrd=off  block_type=slice
  alumode : xbsIndex_r4/Constant  arith_type=Unsigned  const=3  n_bits=4  bin_pt=0  explicit_period=off  period=1  equ=P=C  opselect=C  inp2=PCIN>>17  opr=+  inp1=P  carry=CIN  dbl_ovrd=off  block_type=constant
  alumode0 : xbsIndex_r4/Constant  arith_type=Unsigned  const=0  n_bits=4  bin_pt=0  explicit_period=off  period=1  equ=P=C  opselect=C  inp2=PCIN>>17  opr=+  inp1=P  carry=CIN  dbl_ovrd=off  block_type=constant
      settings: block_version=11.4
  alumode1 : xbsIndex_r4/Constant  arith_type=Unsigned  const=0  n_bits=4  bin_pt=0  explicit_period=off  period=1  equ=P=C  opselect=C  inp2=PCIN>>17  opr=+  inp1=P  carry=CIN  dbl_ovrd=off  block_type=constant
      settings: block_version=11.4
  alumode2 : xbsIndex_r4/Constant  arith_type=Unsigned  const=3  n_bits=4  bin_pt=0  explicit_period=off  period=1  equ=P=C  opselect=C  inp2=PCIN>>17  opr=+  inp1=P  carry=CIN  dbl_ovrd=off  block_type=constant
      settings: block_version=11.4
  alumode3 : xbsIndex_r4/Constant  arith_type=Unsigned  const=0  n_bits=4  bin_pt=0  explicit_period=off  period=1  equ=P=C  opselect=C  inp2=PCIN>>17  opr=+  inp1=P  carry=CIN  dbl_ovrd=off  block_type=constant
      settings: block_version=11.4
  c_to_ri1 : Subsystem  AncestorBlock=casper_library_misc/c_to_ri  mask(c_to_ri){n_bits=a_n_bits, bin_pt=a_bin_pt}
      mask prompts: n_bits "Bit Width"; bin_pt "Binary Point"
      mask help:
      | Outputs real and imaginary components of a complex input.
      | Useful for simplifying interconnects.
      | See also: Real-Imag to Complex (ri_to_c)
      settings: AttributesFormatString=18_17 r/i
      mask Help: eval('xlWeb(''http://casper.berkeley.edu/wiki/C_to_ri'')')
  c_to_ri2 : Subsystem  AncestorBlock=casper_library_misc/c_to_ri  mask(c_to_ri){n_bits=b_n_bits, bin_pt=b_bin_pt}
      mask prompts: n_bits "Bit Width"; bin_pt "Binary Point"
      mask help:
      | Outputs real and imaginary components of a complex input.
      | Useful for simplifying interconnects.
      | See also: Real-Imag to Complex (ri_to_c)
      settings: AttributesFormatString=18_17 r/i
      mask Help: eval('xlWeb(''http://casper.berkeley.edu/wiki/C_to_ri'')')
  c_to_ri3 : Subsystem  AncestorBlock=casper_library_misc/c_to_ri  mask(c_to_ri){n_bits=w_n_bits, bin_pt=w_bin_pt}
      mask prompts: n_bits "Bit Width"; bin_pt "Binary Point"
      mask help:
      | Outputs real and imaginary components of a complex input.
      | Useful for simplifying interconnects.
      | See also: Real-Imag to Complex (ri_to_c)
      settings: AttributesFormatString=18_17 r/i
      mask Help: eval('xlWeb(''http://casper.berkeley.edu/wiki/C_to_ri'')')
  carryin{,0..3} (5 alike) : xbsIndex_r4/Constant  arith_type=Unsigned  const=0  n_bits=1  bin_pt=0  explicit_period=off  period=1  equ=P=C  opselect=C  inp2=PCIN>>17  opr=+  inp1=P  carry=CIN  dbl_ovrd=off  block_type=constant
      carryin0 settings: block_version=11.4
      carryin1 settings: block_version=11.4
      carryin2 settings: block_version=11.4
      carryin3 settings: block_version=11.4
  carryinsel{,0..3} (5 alike) : xbsIndex_r4/Constant  arith_type=Unsigned  const=0  n_bits=3  bin_pt=0  explicit_period=off  period=1  equ=P=C  opselect=C  inp2=PCIN>>17  opr=+  inp1=P  carry=CIN  dbl_ovrd=off  block_type=constant
      carryinsel0 settings: block_version=11.4
      carryinsel1 settings: block_version=11.4
      carryinsel2 settings: block_version=11.4
      carryinsel3 settings: block_version=11.4
  cast_c_im : xbsIndex_r4/Convert  arith_type="Signed  (2's comp)"  n_bits=48  bin_pt=0  quantization=Truncate  overflow=Wrap  en=off  latency=0  dbl_ovrd=off  pipeline=on  block_type=convert
      settings: block_version=11.4
  cast_c_im1 : xbsIndex_r4/Convert  arith_type="Signed  (2's comp)"  n_bits=24  bin_pt=22  quantization=Truncate  overflow=Wrap  en=off  latency=0  dbl_ovrd=off  pipeline=on  block_type=convert
      settings: block_version=10.1.3
  cast_c_re : xbsIndex_r4/Convert  arith_type="Signed  (2's comp)"  n_bits=48  bin_pt=0  quantization=Truncate  overflow=Wrap  en=off  latency=0  dbl_ovrd=off  pipeline=on  block_type=convert
      settings: block_version=11.4
  cast_c_re1 : xbsIndex_r4/Convert  arith_type="Signed  (2's comp)"  n_bits=24  bin_pt=22  quantization=Truncate  overflow=Wrap  en=off  latency=0  dbl_ovrd=off  pipeline=on  block_type=convert
      settings: block_version=10.1.3
  cast_d_im : xbsIndex_r4/Convert  arith_type="Signed  (2's comp)"  n_bits=b_n_bits+w_n_bits + 2  bin_pt=b_bin_pt+w_bin_pt  quantization=Truncate  overflow=Wrap  en=off  latency=0  dbl_ovrd=off  pipeline=on  block_type=convert
      settings: block_version=11.4
  cast_d_im1 : S-Function  LoadFcn=xlBlockLoadCallback(gcbh);  FunctionName=sysgen  Parameters=ptable_  EnableBusSupport=off  mask(Xilinx Type Converter Block){infoedit=Hardware notes: rounding and saturating require hardware resources; truncating and wrapping do not., arith_type_sgadvanced=, arith_type=Signed  (2's comp), n_bits=b_n_bits+w_n_bits + 2, bin_pt=b_bin_pt+w_bin_pt, quantization_sgadvanced=, quantization=Truncate, overflow_sgadvanced=, overflow=Wrap, en_sgadvanced=, en=off, latency=0, dbl_ovrd_sgadvanced=, dbl_ovrd=off, pipeline_sgadvanced=, pipeline=on, xl_use_area_sgadvanced=, xl_use_area=off, xl_area=[0,0,0,0,0,0,0], has_advanced_control=0, sggui_pos=561,83,532,497, block_type=convert, block_version=11.4, sg_icon_stat=45,32,1,1,white,blue,0,edca21da,right,,[ ],[ ], sg_mask_display=|, sg_list_contents=, sg_blockgui_xml=}
      mask sg_mask_display=|
      | fprintf('','COMMENT: begin icon graphics');
      | patch([0 45 45 0 0 ],[0 0 32 32 0 ],[0.77 0.82 0.91 ]);
      | plot([0 45 45 0 0 ],[0 0 32 32 0 ]);
      | patch([13.1 18.88 22.88 26.88 30.88 22.88 17.1 13.1 ],[20.44 20.44 24.44 20.44 24.44 24.44 24.44 20.44 ],[1 1 1 ]);
      | patch([17.1 22.88 18.88 13.1 17.1 ],[16.44 16.44 20.44 20.44 16.44 ],[0.931 0.946 0.973 ]);
      | patch([13.1 18.88 22.88 17.1 13.1 ],[12.44 12.44 16.44 16.44 12.44 ],[1 1 1 ]);
      | patch([17.1 30.88 26.88 22.88 18.88 13.1 17.1 ],[8.44 8.44 12.44 8.44 12.44 12.44 8.44 ],[0.931 0.946 0.973 ]);
      | fprintf('','COMMENT: end icon graphics');
      | fprintf('','COMMENT: begin icon text');
      |
      | color('black');port_label('output',1,'cast');
      | fprintf('','COMMENT: end icon text');
      mask prompts: infoedit ""; arith_type_sgadvanced ""; arith_type "Type"; n_bits "Number of bits"; bin_pt "Binary point"; quantization_sgadvanced ""; overflow_sgadvanced ""; en_sgadvanced ""; en "Provide enable port"; dbl_ovrd_sgadvanced ""; dbl_ovrd "Override with doubles"; pipeline_sgadvanced ""; pipeline "Pipeline for maximum performance"; xl_use_area_sgadvanced ""; xl_use_area "Define FPGA area for resource estimation"; xl_area "FPGA area [slices, FFs, BRAMs, LUTs, IOBs, emb. mults, TBUFs]"; has_advanced_control ""; sggui_pos ""; block_type ""; block_version ""; sg_icon_stat ""; sg_mask_display ""; sg_list_contents ""; sg_blockgui_xml ""
      mask help: Hardware notes: rounding and saturating require hardware resources; truncating and wrapping do not.
      mask init: same as monroe_library/dsp48e_mult_add_pcin/Convert
      settings: CopyFcn=xlBlockMoveCallback(gcbh);  DeleteFcn=xlDestroyGui(gcbh);  ModelCloseFcn=xlDestroyGui(gcbh);  PreSaveFcn=xlBlockPreSaveCallback(gcbh);  PostSaveFcn=xlBlockPostSaveCallback(gcbh);  DestroyFcn=xlDestroyGui(gcbh);  OpenFcn=xlOpenGui(gcbh, 'convert_gui.xml', @convertenablement, -1)  CloseFcn=xlDestroyGui(gcbh);  MoveFcn=xlBlockMoveCallback(gcbh);
      mask Help: eval('');xlDoc('-book','sysgen','-topic','Convert');
      mask TypeOptions arith_type: Boolean | Signed  (2's comp) | Unsigned
      mask TypeOptions quantization: Truncate | Round  (unbiased: +/- Inf) | Round  (unbiased: Even Values)
      mask TypeOptions overflow: Wrap | Saturate | Flag as error
      mask Display:
      | fprintf('','COMMENT: begin icon graphics');
      | patch([0 45 45 0 0 ],[0 0 32 32 0 ],[0.77 0.82 0.91 ]);
      | plot([0 45 45 0 0 ],[0 0 32 32 0 ]);
      | patch([13.1 18.88 22.88 26.88 30.88 22.88 17.1 13.1 ],[20.44 20.44 24.44 20.44 24.44 24.44 24.44 20.44 ],[1 1 1 ]);
      | patch([17.1 22.88 18.88 13.1 17.1 ],[16.44 16.44 20.44 20.44 16.44 ],[0.931 0.946 0.973 ]);
      | patch([13.1 18.88 22.88 17.1 13.1 ],[12.44 12.44 16.44 16.44 12.44 ],[1 1 1 ]);
      | patch([17.1 30.88 26.88 22.88 18.88 13.1 17.1 ],[8.44 8.44 12.44 8.44 12.44 12.44 8.44 ],[0.931 0.946 0.973 ]);
      | fprintf('','COMMENT: end icon graphics');
      | fprintf('','COMMENT: begin icon text');
      | 
      | color('black');port_label('output',1,'cast');
      | fprintf('','COMMENT: end icon text');
  concat_a : xbsIndex_r4/Concat  num_inputs=2  dbl_ovrd=off  block_type=concat
  concat_b : xbsIndex_r4/Concat  num_inputs=2  dbl_ovrd=off  block_type=concat
  delay1 : xbsIndex_r4/Delay  en=off  latency=a_delay  dbl_ovrd=off  reg_retiming=off  block_type=delay
      settings: block_version=11.4
  delay2 : xbsIndex_r4/Delay  en=off  latency=6  dbl_ovrd=off  reg_retiming=off  block_type=delay
      settings: block_version=11.4
  delay3 : xbsIndex_r4/Delay  en=off  latency=a_delay  dbl_ovrd=off  reg_retiming=off  block_type=delay
      settings: block_version=11.4
  delay4 : xbsIndex_r4/Delay  en=off  latency=2*apbw_delay  dbl_ovrd=off  reg_retiming=off  block_type=delay
      settings: block_version=11.4
  delay5 : xbsIndex_r4/Delay  en=off  latency=3+a_delay  dbl_ovrd=off  reg_retiming=off  block_type=delay
      settings: block_version=11.4
  delay6 : xbsIndex_r4/Delay  en=off  latency=3+a_delay  dbl_ovrd=off  reg_retiming=off  block_type=delay
      settings: block_version=11.4
  delay7 : xbsIndex_r4/Delay  en=off  latency=2*apbw_delay  dbl_ovrd=off  reg_retiming=off  block_type=delay
      settings: block_version=11.4
  dsp_AmBW : xbsIndex_r4/DSP48E  use_a=Direct from A Port  use_b=Direct from B Port  reset_preg=off  pattern_from_creg=off  pattern='000000000000'  mask_from_creg=off  pattern_mask='3FFFFFFFFFFF'  sel_rounding_mask=Select mask  use_op=off  use_creg=on  rst_all=off  en_all=off  use_pcin=on  use_carrycascin=off  use_multsignin=off  use_carryout=off  use_patterndetect=off  use_patternbdetect=off  use_overflow=off  use_underflow=off  use_acout=off  use_bcout=off  use_pcout=off  use_multsignout=off  use_carrycascout=off  pipeline_a=1  pipeline_b=1  pipeline_acout=1  pipeline_bcout=1  pipeline_c=on  pipeline_p=on  pipeline_mult=on  pipeline_opmode=on  pipeline_alumode=on  pipeline_carryin=on  pipeline_carryinsel=on  rst_a=off  rst_b=off  rst_c=off  rst_mult=off  rst_p=off  rst_carry_in=off  rst_alumode=off  rst_ctrl=off  en_a1=off  en_a2=off  en_b1=off  en_b2=off  en_c=off  en_mult=off  en_p=off  en_carry_in=off  en_alumode=off  en_multcarryin=off  en_ctrl=off  use_synth_model=off  addsub_mode=TWO24  xl_useadderonly=on  block_type=dsp48e
      settings: block_version=10.1.3
  dsp_ApBW_im_1 : xbsIndex_r4/DSP48E  use_a=Direct from A Port  use_b=Direct from B Port  reset_preg=off  pattern_from_creg=off  pattern='000000000000'  mask_from_creg=off  pattern_mask='3FFFFFFFFFFF'  sel_rounding_mask=Select mask  use_op=off  use_creg=off  rst_all=off  en_all=off  use_pcin=on  use_carrycascin=off  use_multsignin=off  use_carryout=off  use_patterndetect=off  use_patternbdetect=off  use_overflow=off  use_underflow=off  use_acout=off  use_bcout=off  use_pcout=on  use_multsignout=off  use_carrycascout=off  pipeline_a=2  pipeline_b=2  pipeline_acout=1  pipeline_bcout=1  pipeline_c=on  pipeline_p=on  pipeline_mult=on  pipeline_opmode=on  pipeline_alumode=on  pipeline_carryin=on  pipeline_carryinsel=on  rst_a=off  rst_b=off  rst_c=off  rst_mult=off  rst_p=off  rst_carry_in=off  rst_alumode=off  rst_ctrl=off  en_a1=off  en_a2=off  en_b1=off  en_b2=off  en_c=off  en_mult=off  en_p=off  en_carry_in=off  en_alumode=off  en_multcarryin=off  en_ctrl=off  use_synth_model=off  addsub_mode=ONE48  xl_useadderonly=off  block_type=dsp48e
      settings: block_version=11.4
  dsp_ApBW_im_2 : xbsIndex_r4/DSP48E  use_a=Direct from A Port  use_b=Direct from B Port  reset_preg=off  pattern_from_creg=off  pattern='000000000000'  mask_from_creg=off  pattern_mask='3FFFFFFFFFFF'  sel_rounding_mask=Select mask  use_op=off  use_creg=on  rst_all=off  en_all=off  use_pcin=off  use_carrycascin=off  use_multsignin=off  use_carryout=off  use_patterndetect=off  use_patternbdetect=off  use_overflow=off  use_underflow=off  use_acout=off  use_bcout=off  use_pcout=on  use_multsignout=off  use_carrycascout=off  pipeline_a=1  pipeline_b=1  pipeline_acout=1  pipeline_bcout=1  pipeline_c=on  pipeline_p=on  pipeline_mult=on  pipeline_opmode=on  pipeline_alumode=on  pipeline_carryin=on  pipeline_carryinsel=on  rst_a=off  rst_b=off  rst_c=off  rst_mult=off  rst_p=off  rst_carry_in=off  rst_alumode=off  rst_ctrl=off  en_a1=off  en_a2=off  en_b1=off  en_b2=off  en_c=off  en_mult=off  en_p=off  en_carry_in=off  en_alumode=off  en_multcarryin=off  en_ctrl=off  use_synth_model=off  addsub_mode=ONE48  xl_useadderonly=off  block_type=dsp48e
      settings: block_version=11.4
  dsp_ApBW_re_1 : xbsIndex_r4/DSP48E  use_a=Direct from A Port  use_b=Direct from B Port  reset_preg=off  pattern_from_creg=off  pattern='000000000000'  mask_from_creg=off  pattern_mask='3FFFFFFFFFFF'  sel_rounding_mask=Select mask  use_op=off  use_creg=off  rst_all=off  en_all=off  use_pcin=on  use_carrycascin=off  use_multsignin=off  use_carryout=off  use_patterndetect=off  use_patternbdetect=off  use_overflow=off  use_underflow=off  use_acout=off  use_bcout=off  use_pcout=off  use_multsignout=off  use_carrycascout=off  pipeline_a=2  pipeline_b=2  pipeline_acout=1  pipeline_bcout=1  pipeline_c=on  pipeline_p=on  pipeline_mult=on  pipeline_opmode=on  pipeline_alumode=on  pipeline_carryin=on  pipeline_carryinsel=on  rst_a=off  rst_b=off  rst_c=off  rst_mult=off  rst_p=off  rst_carry_in=off  rst_alumode=off  rst_ctrl=off  en_a1=off  en_a2=off  en_b1=off  en_b2=off  en_c=off  en_mult=off  en_p=off  en_carry_in=off  en_alumode=off  en_multcarryin=off  en_ctrl=off  use_synth_model=off  addsub_mode=ONE48  xl_useadderonly=off  block_type=dsp48e
      settings: block_version=11.4
  dsp_ApBW_re_2 : xbsIndex_r4/DSP48E  use_a=Direct from A Port  use_b=Direct from B Port  reset_preg=off  pattern_from_creg=off  pattern='000000000000'  mask_from_creg=off  pattern_mask='3FFFFFFFFFFF'  sel_rounding_mask=Select mask  use_op=off  use_creg=on  rst_all=off  en_all=off  use_pcin=off  use_carrycascin=off  use_multsignin=off  use_carryout=off  use_patterndetect=off  use_patternbdetect=off  use_overflow=off  use_underflow=off  use_acout=off  use_bcout=off  use_pcout=on  use_multsignout=off  use_carrycascout=off  pipeline_a=1  pipeline_b=1  pipeline_acout=1  pipeline_bcout=1  pipeline_c=on  pipeline_p=on  pipeline_mult=on  pipeline_opmode=on  pipeline_alumode=on  pipeline_carryin=on  pipeline_carryinsel=on  rst_a=off  rst_b=off  rst_c=off  rst_mult=off  rst_p=off  rst_carry_in=off  rst_alumode=off  rst_ctrl=off  en_a1=off  en_a2=off  en_b1=off  en_b2=off  en_c=off  en_mult=off  en_p=off  en_carry_in=off  en_alumode=off  en_multcarryin=off  en_ctrl=off  use_synth_model=off  addsub_mode=ONE48  xl_useadderonly=off  block_type=dsp48e
      settings: block_version=11.4
  opmode : xbsIndex_r4/Constant  arith_type=Unsigned  const=51  n_bits=7  bin_pt=0  explicit_period=off  period=1  equ=P=C  opselect=C  inp2=PCIN>>17  opr=+  inp1=P  carry=CIN  dbl_ovrd=off  block_type=constant
  opmode0 : xbsIndex_r4/Constant  arith_type=Unsigned  const=53  n_bits=7  bin_pt=0  explicit_period=off  period=1  equ=P=C  opselect=C  inp2=PCIN>>17  opr=+  inp1=P  carry=CIN  dbl_ovrd=off  block_type=constant
      settings: block_version=11.4
  opmode1 : xbsIndex_r4/Constant  arith_type=Unsigned  const=21  n_bits=7  bin_pt=0  explicit_period=off  period=1  equ=P=C  opselect=C  inp2=PCIN>>17  opr=+  inp1=P  carry=CIN  dbl_ovrd=off  block_type=constant
      settings: block_version=11.4
  opmode2 : xbsIndex_r4/Constant  arith_type=Unsigned  const=53  n_bits=7  bin_pt=0  explicit_period=off  period=1  equ=P=C  opselect=C  inp2=PCIN>>17  opr=+  inp1=P  carry=CIN  dbl_ovrd=off  block_type=constant
      settings: block_version=11.4
  opmode3 : xbsIndex_r4/Constant  arith_type=Unsigned  const=21  n_bits=7  bin_pt=0  explicit_period=off  period=1  equ=P=C  opselect=C  inp2=PCIN>>17  opr=+  inp1=P  carry=CIN  dbl_ovrd=off  block_type=constant
      settings: block_version=11.4
  realign_a_im : xbsIndex_r4/Convert  arith_type="Signed  (2's comp)"  n_bits=b_n_bits  bin_pt=b_bin_pt  quantization=Truncate  overflow=Wrap  en=off  latency=0  dbl_ovrd=off  pipeline=on  block_type=convert
      settings: block_version=11.4
  realign_a_im1 : xbsIndex_r4/Convert  arith_type="Signed  (2's comp)"  n_bits=24  bin_pt=22  quantization=Truncate  overflow=Wrap  en=off  latency=0  dbl_ovrd=off  pipeline=on  block_type=convert
      settings: block_version=10.1.3
  realign_a_re : xbsIndex_r4/Convert  arith_type="Signed  (2's comp)"  n_bits=b_n_bits  bin_pt=b_bin_pt  quantization=Truncate  overflow=Wrap  en=off  latency=0  dbl_ovrd=off  pipeline=on  block_type=convert
      settings: block_version=11.4
  realign_a_re1 : xbsIndex_r4/Convert  arith_type="Signed  (2's comp)"  n_bits=24  bin_pt=22  quantization=Truncate  overflow=Wrap  en=off  latency=0  dbl_ovrd=off  pipeline=on  block_type=convert
      settings: block_version=10.1.3
  realign_b_im : xbsIndex_r4/Convert  arith_type="Signed  (2's comp)"  n_bits=w_n_bits  bin_pt=w_bin_pt  quantization=Truncate  overflow=Wrap  en=off  latency=0  dbl_ovrd=off  pipeline=on  block_type=convert
      settings: block_version=11.4
  realign_b_im1 : xbsIndex_r4/Convert  arith_type="Signed  (2's comp)"  n_bits=24  bin_pt=22  quantization=Truncate  overflow=Wrap  en=off  latency=0  dbl_ovrd=off  pipeline=on  block_type=convert
      settings: block_version=10.1.3
  realign_b_re : xbsIndex_r4/Convert  arith_type="Signed  (2's comp)"  n_bits=w_n_bits  bin_pt=w_bin_pt  quantization=Truncate  overflow=Wrap  en=off  latency=0  dbl_ovrd=off  pipeline=on  block_type=convert
      settings: block_version=11.4
  realign_b_re1 : xbsIndex_r4/Convert  arith_type="Signed  (2's comp)"  n_bits=24  bin_pt=22  quantization=Truncate  overflow=Wrap  en=off  latency=0  dbl_ovrd=off  pipeline=on  block_type=convert
      settings: block_version=10.1.3
  realign_c_im : xbsIndex_r4/Convert  arith_type="Signed  (2's comp)"  n_bits=48  bin_pt=b_bin_pt+w_bin_pt  quantization=Truncate  overflow=Wrap  en=off  latency=0  dbl_ovrd=off  pipeline=on  block_type=convert
      settings: block_version=11.4
  realign_c_re : xbsIndex_r4/Convert  arith_type="Signed  (2's comp)"  n_bits=48  bin_pt=b_bin_pt+w_bin_pt  quantization=Truncate  overflow=Wrap  en=off  latency=0  dbl_ovrd=off  pipeline=on  block_type=convert
      settings: block_version=11.4
  reinterp_a_im : xbsIndex_r4/Reinterpret  force_arith_type=on  arith_type="Signed  (2's comp)"  force_bin_pt=on  bin_pt=0  block_type=reinterpret
      settings: infoedit="Changes signal type without altering the binary representation.   You can changed the signal between signed and unsigned, and relocate the binary point.<br><br>Hardware notes: In hardware this block costs nothing.<br><br>Example:  Suppose the input is 6 bits wide, signed, with 2 fractional bits, and the output is forced to unsigned with 0 fractional bits.  Then an input of -2.0 (1110.00 in binary 2's complement) becomes an output of 56 (111000 in binary)."
  reinterp_a_im1 : xbsIndex_r4/Reinterpret  force_arith_type=on  arith_type=Unsigned  force_bin_pt=on  bin_pt=0  block_type=reinterpret
      settings: infoedit="Changes signal type without altering the binary representation.   You can changed the signal between signed and unsigned, and relocate the binary point.<br><br>Hardware notes: In hardware this block costs nothing.<br><br>Example:  Suppose the input is 6 bits wide, signed, with 2 fractional bits, and the output is forced to unsigned with 0 fractional bits.  Then an input of -2.0 (1110.00 in binary 2's complement) becomes an output of 56 (111000 in binary)."  block_version=10.1.3
  reinterp_a_re : xbsIndex_r4/Reinterpret  force_arith_type=on  arith_type="Signed  (2's comp)"  force_bin_pt=on  bin_pt=0  block_type=reinterpret
      settings: infoedit="Changes signal type without altering the binary representation.   You can changed the signal between signed and unsigned, and relocate the binary point.<br><br>Hardware notes: In hardware this block costs nothing.<br><br>Example:  Suppose the input is 6 bits wide, signed, with 2 fractional bits, and the output is forced to unsigned with 0 fractional bits.  Then an input of -2.0 (1110.00 in binary 2's complement) becomes an output of 56 (111000 in binary)."
  reinterp_a_re1 : xbsIndex_r4/Reinterpret  force_arith_type=on  arith_type=Unsigned  force_bin_pt=on  bin_pt=0  block_type=reinterpret
      settings: infoedit="Changes signal type without altering the binary representation.   You can changed the signal between signed and unsigned, and relocate the binary point.<br><br>Hardware notes: In hardware this block costs nothing.<br><br>Example:  Suppose the input is 6 bits wide, signed, with 2 fractional bits, and the output is forced to unsigned with 0 fractional bits.  Then an input of -2.0 (1110.00 in binary 2's complement) becomes an output of 56 (111000 in binary)."  block_version=10.1.3
  reinterp_b_im : xbsIndex_r4/Reinterpret  force_arith_type=on  arith_type="Signed  (2's comp)"  force_bin_pt=on  bin_pt=0  block_type=reinterpret
      settings: infoedit="Changes signal type without altering the binary representation.   You can changed the signal between signed and unsigned, and relocate the binary point.<br><br>Hardware notes: In hardware this block costs nothing.<br><br>Example:  Suppose the input is 6 bits wide, signed, with 2 fractional bits, and the output is forced to unsigned with 0 fractional bits.  Then an input of -2.0 (1110.00 in binary 2's complement) becomes an output of 56 (111000 in binary)."
  reinterp_b_im1 : xbsIndex_r4/Reinterpret  force_arith_type=on  arith_type=Unsigned  force_bin_pt=on  bin_pt=0  block_type=reinterpret
      settings: infoedit="Changes signal type without altering the binary representation.   You can changed the signal between signed and unsigned, and relocate the binary point.<br><br>Hardware notes: In hardware this block costs nothing.<br><br>Example:  Suppose the input is 6 bits wide, signed, with 2 fractional bits, and the output is forced to unsigned with 0 fractional bits.  Then an input of -2.0 (1110.00 in binary 2's complement) becomes an output of 56 (111000 in binary)."  block_version=10.1.3
  reinterp_b_re : xbsIndex_r4/Reinterpret  force_arith_type=on  arith_type="Signed  (2's comp)"  force_bin_pt=on  bin_pt=0  block_type=reinterpret
      settings: infoedit="Changes signal type without altering the binary representation.   You can changed the signal between signed and unsigned, and relocate the binary point.<br><br>Hardware notes: In hardware this block costs nothing.<br><br>Example:  Suppose the input is 6 bits wide, signed, with 2 fractional bits, and the output is forced to unsigned with 0 fractional bits.  Then an input of -2.0 (1110.00 in binary 2's complement) becomes an output of 56 (111000 in binary)."
  reinterp_b_re1 : xbsIndex_r4/Reinterpret  force_arith_type=on  arith_type=Unsigned  force_bin_pt=on  bin_pt=0  block_type=reinterpret
      settings: infoedit="Changes signal type without altering the binary representation.   You can changed the signal between signed and unsigned, and relocate the binary point.<br><br>Hardware notes: In hardware this block costs nothing.<br><br>Example:  Suppose the input is 6 bits wide, signed, with 2 fractional bits, and the output is forced to unsigned with 0 fractional bits.  Then an input of -2.0 (1110.00 in binary 2's complement) becomes an output of 56 (111000 in binary)."  block_version=10.1.3
  reinterp_c_im : xbsIndex_r4/Reinterpret  force_arith_type=on  arith_type="Signed  (2's comp)"  force_bin_pt=on  bin_pt=0  block_type=reinterpret
      settings: infoedit="Changes signal type without altering the binary representation.   You can changed the signal between signed and unsigned, and relocate the binary point.<br><br>Hardware notes: In hardware this block costs nothing.<br><br>Example:  Suppose the input is 6 bits wide, signed, with 2 fractional bits, and the output is forced to unsigned with 0 fractional bits.  Then an input of -2.0 (1110.00 in binary 2's complement) becomes an output of 56 (111000 in binary)."
  reinterp_c_im1 : xbsIndex_r4/Reinterpret  force_arith_type=on  arith_type="Signed  (2's comp)"  force_bin_pt=on  bin_pt=22  block_type=reinterpret
      settings: infoedit="Changes signal type without altering the binary representation.   You can changed the signal between signed and unsigned, and relocate the binary point.<br><br>Hardware notes: In hardware this block costs nothing.<br><br>Example:  Suppose the input is 6 bits wide, signed, with 2 fractional bits, and the output is forced to unsigned with 0 fractional bits.  Then an input of -2.0 (1110.00 in binary 2's complement) becomes an output of 56 (111000 in binary)."  block_version=10.1.3
  reinterp_c_re : xbsIndex_r4/Reinterpret  force_arith_type=on  arith_type="Signed  (2's comp)"  force_bin_pt=on  bin_pt=0  block_type=reinterpret
      settings: infoedit="Changes signal type without altering the binary representation.   You can changed the signal between signed and unsigned, and relocate the binary point.<br><br>Hardware notes: In hardware this block costs nothing.<br><br>Example:  Suppose the input is 6 bits wide, signed, with 2 fractional bits, and the output is forced to unsigned with 0 fractional bits.  Then an input of -2.0 (1110.00 in binary 2's complement) becomes an output of 56 (111000 in binary)."
  reinterp_c_re1 : xbsIndex_r4/Reinterpret  force_arith_type=on  arith_type="Signed  (2's comp)"  force_bin_pt=on  bin_pt=22  block_type=reinterpret
      settings: infoedit="Changes signal type without altering the binary representation.   You can changed the signal between signed and unsigned, and relocate the binary point.<br><br>Hardware notes: In hardware this block costs nothing.<br><br>Example:  Suppose the input is 6 bits wide, signed, with 2 fractional bits, and the output is forced to unsigned with 0 fractional bits.  Then an input of -2.0 (1110.00 in binary 2's complement) becomes an output of 56 (111000 in binary)."  block_version=10.1.3
  reinterp_d_im : xbsIndex_r4/Reinterpret  force_arith_type=on  arith_type="Signed  (2's comp)"  force_bin_pt=on  bin_pt=b_bin_pt+w_bin_pt  block_type=reinterpret
      settings: infoedit="Changes signal type without altering the binary representation.   You can changed the signal between signed and unsigned, and relocate the binary point.<br><br>Hardware notes: In hardware this block costs nothing.<br><br>Example:  Suppose the input is 6 bits wide, signed, with 2 fractional bits, and the output is forced to unsigned with 0 fractional bits.  Then an input of -2.0 (1110.00 in binary 2's complement) becomes an output of 56 (111000 in binary)."
  reinterp_d_re : xbsIndex_r4/Reinterpret  force_arith_type=on  arith_type="Signed  (2's comp)"  force_bin_pt=on  bin_pt=b_bin_pt+w_bin_pt  block_type=reinterpret
      settings: infoedit="Changes signal type without altering the binary representation.   You can changed the signal between signed and unsigned, and relocate the binary point.<br><br>Hardware notes: In hardware this block costs nothing.<br><br>Example:  Suppose the input is 6 bits wide, signed, with 2 fractional bits, and the output is forced to unsigned with 0 fractional bits.  Then an input of -2.0 (1110.00 in binary 2's complement) becomes an output of 56 (111000 in binary)."
  slice_c_im : xbsIndex_r4/Slice  nbits=24  boolean_output=off  mode=Lower Bit Location + Width  bit1=0  base1=MSB of Input  bit0=0  base0=LSB of Input  dbl_ovrd=off  block_type=slice
  slice_c_re : xbsIndex_r4/Slice  nbits=24  boolean_output=off  mode=Lower Bit Location + Width  bit1=0  base1=MSB of Input  bit0=24  base0=LSB of Input  dbl_ovrd=off  block_type=slice
  a+bw : Outport
  a-bw : Outport  Port=2
  sync_out : Outport  Port=3
  wires:
  [b_im] -> realign_a_im/1
  c_to_ri3/2(im) -> [w_im]
  c_to_ri3/1(re) -> [w_re]
  w/1 -> c_to_ri3/1(c)
  c_to_ri2/2(im) -> [b_im]
  c_to_ri2/1(re) -> [b_re]
  b/1 -> c_to_ri2/1(c)
  c_to_ri1/2(im) -> [a_im]
  c_to_ri1/1(re) -> [a_re]
  a/1 -> c_to_ri1/1(c)
  delay2/1 -> sync_out/1
  sync/1 -> delay2/1
  reinterp_a_re1/1 -> concat_a/1
  reinterp_b_im1/1 -> concat_b/2
  reinterp_b_re1/1 -> concat_b/1
  reinterp_a_im1/1 -> concat_a/2
  concat_b/1 -> Slice_A/1, Slice_B/1
  Reinterpret_C/1 -> dsp_AmBW/3
  reinterp_c_im1/1 -> cast_c_im1/1
  reinterp_c_re1/1 -> cast_c_re1/1
  slice_c_im/1 -> reinterp_c_im1/1
  slice_c_re/1 -> reinterp_c_re1/1
  dsp_AmBW/1 -> slice_c_re/1, slice_c_im/1
  Slice_A/1 -> Reinterpret_A/1
  Slice_B/1 -> Reinterpret_B/1
  concat_a/1 -> Reinterpret_C/1
  Reinterpret_B/1 -> dsp_AmBW/2
  Reinterpret_A/1 -> dsp_AmBW/1
  realign_a_re1/1 -> reinterp_a_re1/1
  realign_a_im1/1 -> reinterp_a_im1/1
  realign_b_re1/1 -> reinterp_b_re1/1
  realign_b_im1/1 -> reinterp_b_im1/1
  reinterp_a_im/1 -> Convert/1
  [a_im] -> delay6/1
  delay6/1 -> Scale1/1
  delay5/1 -> Scale/1
  [a_re] -> delay5/1
  Scale1/1 -> realign_a_im1/1
  Scale/1 -> realign_a_re1/1
  [b_re] -> realign_a_re/1
  delay1/1 -> realign_c_im/1
  [a_im] -> delay1/1
  delay3/1 -> realign_c_re/1
  [a_re] -> delay3/1
  cast_d_im/1 -> delay4/1, realign_b_im1/1
  cast_d_im1/1 -> realign_b_re1/1, delay7/1
  [w_im] -> realign_b_im/1
  [w_re] -> realign_b_re/1
  reinterp_d_re/1 -> cast_d_im1/1
  dsp_ApBW_im_1/1 -> reinterp_d_im/1
  realign_b_im/1 -> reinterp_b_im/1
  realign_a_im/1 -> reinterp_a_im/1
  opmode3/1 -> dsp_ApBW_re_1/4
  opmode2/1 -> dsp_ApBW_re_2/4
  opmode1/1 -> dsp_ApBW_im_1/4
  opmode0/1 -> dsp_ApBW_im_2/4
  carryinsel3/1 -> dsp_ApBW_re_1/7
  carryinsel2/1 -> dsp_ApBW_re_2/7
  carryinsel1/1 -> dsp_ApBW_im_1/7
  carryinsel0/1 -> dsp_ApBW_im_2/7
  carryin3/1 -> dsp_ApBW_re_1/6
  carryin2/1 -> dsp_ApBW_re_2/6
  carryin1/1 -> dsp_ApBW_im_1/6
  carryin0/1 -> dsp_ApBW_im_2/6
  alumode3/1 -> dsp_ApBW_re_1/5
  alumode2/1 -> dsp_ApBW_re_2/5
  alumode1/1 -> dsp_ApBW_im_1/5
  alumode0/1 -> dsp_ApBW_im_2/5
  dsp_ApBW_re_2/2 -> dsp_ApBW_re_1/3
  Convert2/1 -> dsp_ApBW_im_1/1, dsp_ApBW_re_1/1
  cast_c_re/1 -> dsp_ApBW_re_2/3
  Convert/1 -> dsp_ApBW_im_2/1, dsp_ApBW_re_2/1
  dsp_ApBW_im_2/2 -> dsp_ApBW_im_1/3
  cast_c_im/1 -> dsp_ApBW_im_2/3
  reinterp_c_im/1 -> cast_c_im/1
  realign_c_im/1 -> reinterp_c_im/1
  reinterp_c_re/1 -> cast_c_re/1
  realign_c_re/1 -> reinterp_c_re/1
  Convert6/1 -> dsp_ApBW_im_2/2
  Convert7/1 -> dsp_ApBW_im_1/2
  Convert3/1 -> dsp_ApBW_re_2/2
  Convert4/1 -> dsp_ApBW_re_1/2
  realign_a_re/1 -> reinterp_a_re/1
  realign_b_re/1 -> reinterp_b_re/1
  reinterp_d_im/1 -> cast_d_im/1
  dsp_ApBW_re_1/1 -> reinterp_d_re/1
  reinterp_b_re/1 -> Convert6/1, Convert4/1
  reinterp_b_im/1 -> Convert7/1, Convert3/1
  reinterp_a_re/1 -> Convert2/1
  opmode/1 -> dsp_AmBW/5
  alumode/1 -> dsp_AmBW/6
  carryin/1 -> dsp_AmBW/7
  carryinsel/1 -> dsp_AmBW/8
  dsp_ApBW_im_1/2 -> dsp_AmBW/4
  Scale5/1 -> Convert9/1  "xlsub2_Scale3_out1"
  Scale4/1 -> Convert8/1  "xlsub2_Scale2_out1"
  Reinterpret3/1 -> Concat1/2  "xlsub2_Reinterpret3_out1"
  Convert9/1 -> Reinterpret3/1  "xlsub2_Convert3_out1"
  Reinterpret2/1 -> Concat1/1  "xlsub2_Reinterpret2_out1"
  Convert8/1 -> Reinterpret2/1  "xlsub2_Convert2_out1"
  Concat1/1 -> a-bw/1
  cast_c_im1/1 -> Scale5/1
  cast_c_re1/1 -> Scale4/1
  Scale7/1 -> Convert11/1  "xlsub2_Scale3_out1"
  Scale6/1 -> Convert10/1  "xlsub2_Scale2_out1"
  Reinterpret5/1 -> Concat2/2  "xlsub2_Reinterpret3_out1"
  Convert11/1 -> Reinterpret5/1  "xlsub2_Convert3_out1"
  Reinterpret4/1 -> Concat2/1  "xlsub2_Reinterpret2_out1"
  Convert10/1 -> Reinterpret4/1  "xlsub2_Convert2_out1"
  delay4/1 -> Scale7/1
  delay7/1 -> Scale6/1
  Concat2/1 -> a+bw/1
